simulink model "volo_agcdc_pipelined"  (R2012b)
settings: Solver=ode45  StartTime=0.0  StopTime=1000  RelTol=1e-3
PreLoadFcn:
  | volo_agcdc_init
InitFcn:
  | volo_agcdc_init
StartFcn:
  | volo_agcdc_init
values from neighbouring files (symbols this model uses):
  agc_idleState = 0    [volo_agcdc_init.m]
  agc_numAddrBits = agc_numOutputs + agc_numStateBits    [volo_agcdc_init.m]
  regDCRemoval_AvgLength = 64    [volo_agcdc_init.m]
  regSatDet_NumSamples = 16    [volo_agcdc_init.m]
undefined symbols (not defined in the file or in its folder): gcbh, xlBlockLoadCallback, xlGetNormalizedPeriod
libraries: xbsIndex_r4 x681, xbsEDKLib_r4 x1
(part 5 of 7)

== system volo_agcdc_pipelined/Ext_PktDet_Delay ==
  Set : Inport
  Rst : Inport  Port=2
  "Ext Pkt Det Delay " : Subsystem
  S-R Latch2 : Subsystem
  Out : Outport
  wires:
  S-R Latch2/1(Q) -> "Ext Pkt Det Delay "/1(In)  "ext detect pending"
  Rst/1 -> S-R Latch2/2(R)
  Set/1 -> S-R Latch2/1(S)
  "Ext Pkt Det Delay "/1(Out) -> Out/1  "xternal detection"

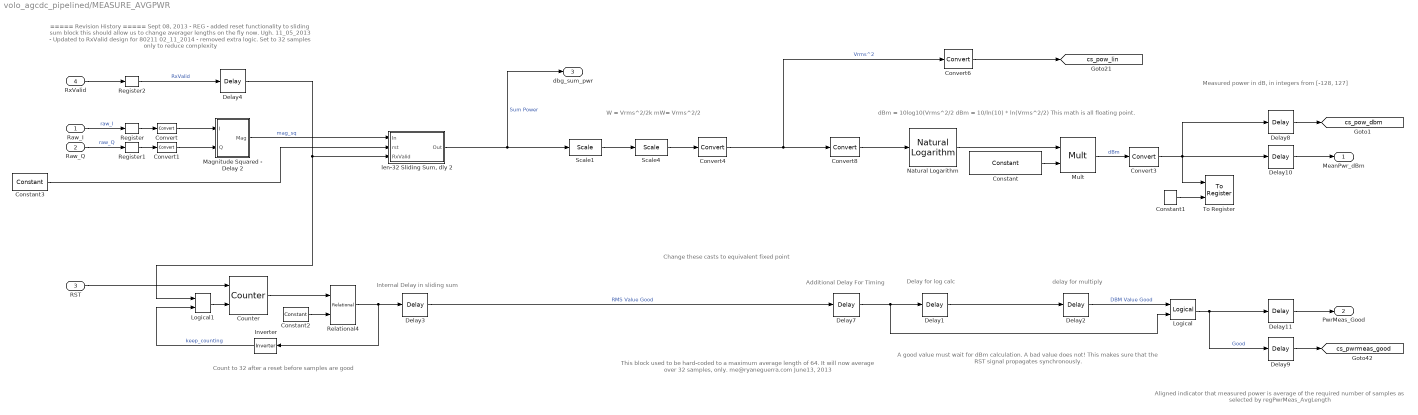
== system volo_agcdc_pipelined/MEASURE_AVGPWR ==
  note: delay for multiply
  note: Delay for log calc
  note: Count to 32 after a reset before samples are good
  note: Change these casts to equivalent fixed point
  note: Additional Delay For Timing
  note: Internal Delay in sliding sum
  note: ===== Revision History =====
      | Sept 08, 2013 - REG - added reset functionality to sliding sum block
      | this should allow us to change averager lengths on the fly now. Ugh.
      | 11_05_2013 - Updated to RxValid design for 80211
      | 02_11_2014 - removed extra logic. Set to 32 samples only to reduce complexity
  note: A good value must wait for dBm calculation.
      | A bad value does not! This makes sure that
      | the RST signal propagates synchronously.
  note: Aligned indicator that
      | measured power is average
      | of the required number
      | of samples as selected
      | by regPwrMeas_AvgLength
  note: Measured power in dB,
      | in  integers from
      | [-128, 127]
  note: dBm = 10log10(Vrms^2/2
      | dBm = 10/ln(10) * ln(Vrms^2/2)
      | This math is all floating point.
  note: W = Vrms^2/2k
      | mW= Vrms^2/2
  note: This block used to be hard-coded to a maximum average length of 64.
      | It will now average over 32 samples, only.
      | me@ryaneguerra.com
      | June13, 2013
  Raw_I : Inport
  Raw_Q : Inport  Port=2
  RST : Inport  Port=3
  RxValid : Inport  Port=4
  Constant : xbsIndex_r4/Constant  const=10/log(10)  gui_display_data_type=Floating-point  arith_type=Floating-point  n_bits=18  bin_pt=14  preci_type=Single  exp_width=8  frac_width=24  explicit_period=on  period=1  equ=P=C  opselect=C  inp2=PCIN>>17  opr=+  inp1=P  carry=CIN  dbl_ovrd=off  block_type=constant
  Constant1 : xbsIndex_r4/Constant  const=1  gui_display_data_type=Boolean  arith_type=Boolean  n_bits=18  bin_pt=14  preci_type=Single  exp_width=8  frac_width=24  explicit_period=on  period=1  equ=P=C  opselect=C  inp2=PCIN>>17  opr=+  inp1=P  carry=CIN  dbl_ovrd=off  block_type=constant
  Constant2 : xbsIndex_r4/Constant  const=32  gui_display_data_type=Fixed-point  arith_type=Unsigned  n_bits=6  bin_pt=0  preci_type=Single  exp_width=8  frac_width=24  explicit_period=on  period=1  equ=P=C  opselect=C  inp2=PCIN>>17  opr=+  inp1=P  carry=CIN  dbl_ovrd=off  block_type=constant
  Constant3 : xbsIndex_r4/Constant  const=0  gui_display_data_type=Boolean  arith_type=Boolean  n_bits=16  bin_pt=14  preci_type=Single  exp_width=8  frac_width=24  explicit_period=on  period=1  equ=P=C  opselect=C  inp2=PCIN>>17  opr=+  inp1=P  carry=CIN  dbl_ovrd=off  block_type=constant
  Convert : xbsIndex_r4/Convert  gui_display_data_type=Fixed-point  arith_type="Signed  (2's comp)"  n_bits=12  bin_pt=11  float_type=Single  exp_bits=8  fraction_bits=24  quantization=Truncate  overflow=Wrap  en=off  latency=0  dbl_ovrd=off  pipeline=off  block_type=convert
  Convert1 : xbsIndex_r4/Convert  gui_display_data_type=Fixed-point  arith_type="Signed  (2's comp)"  n_bits=12  bin_pt=11  float_type=Single  exp_bits=8  fraction_bits=24  quantization=Truncate  overflow=Wrap  en=off  latency=0  dbl_ovrd=off  pipeline=off  block_type=convert
  Convert3 : xbsIndex_r4/Convert  gui_display_data_type=Fixed-point  arith_type="Signed  (2's comp)"  n_bits=9  bin_pt=0  float_type=Single  exp_bits=8  fraction_bits=24  quantization="Round  (unbiased: +/- Inf)"  overflow=Saturate  en=off  latency=0  dbl_ovrd=off  pipeline=off  block_type=convert
  Convert4 : xbsIndex_r4/Convert  gui_display_data_type=Fixed-point  arith_type="Signed  (2's comp)"  n_bits=34  bin_pt=22  float_type=Single  exp_bits=8  fraction_bits=24  quantization=Truncate  overflow=Wrap  en=off  latency=0  dbl_ovrd=off  pipeline=off  block_type=convert
  Convert6 : xbsIndex_r4/Convert  gui_display_data_type=Fixed-point  arith_type="Signed  (2's comp)"  n_bits=32  bin_pt=15  float_type=Single  exp_bits=8  fraction_bits=24  quantization="Round  (unbiased: +/- Inf)"  overflow=Saturate  en=off  latency=0  dbl_ovrd=off  pipeline=off  block_type=convert
  Convert8 : xbsIndex_r4/Convert  gui_display_data_type=Floating-point  arith_type=Floating-point  n_bits=34  bin_pt=22  float_type=Single  exp_bits=8  fraction_bits=24  quantization=Truncate  overflow=Wrap  en=off  latency=3  dbl_ovrd=off  pipeline=on  block_type=convert
  Counter : xbsIndex_r4/Counter  cnt_type=Free Running  cnt_to=10  operation=Up  start_count=0  cnt_by_val=1  arith_type=Unsigned  n_bits=10  bin_pt=0  load_pin=off  rst=on  en=on  explicit_period=on  period=1  dbl_ovrd=off  use_behavioral_HDL=off  implementation=Fabric  block_type=counter
  Delay1 : xbsIndex_r4/Delay  rst=off  infoeditControl=Selection of Reset will increase slice count due to use of real FFs and instead of SRLs  en=off  latency=6  dbl_ovrd=off  reg_retiming=off  block_type=delay
  Delay{8..11} (4 alike) : xbsIndex_r4/Delay  rst=off  infoeditControl=Selection of Reset will increase slice count due to use of real FFs and instead of SRLs  en=off  latency=1  dbl_ovrd=off  reg_retiming=off  block_type=delay
  Delay2 : xbsIndex_r4/Delay  rst=off  infoeditControl=Selection of Reset will increase slice count due to use of real FFs and instead of SRLs  en=off  latency=6  dbl_ovrd=off  reg_retiming=off  block_type=delay
  Delay3 : xbsIndex_r4/Delay  rst=off  infoeditControl=Selection of Reset will increase slice count due to use of real FFs and instead of SRLs  en=off  latency=2  dbl_ovrd=off  reg_retiming=off  block_type=delay
  Delay4 : xbsIndex_r4/Delay  rst=off  infoeditControl=Selection of Reset will increase slice count due to use of real FFs and instead of SRLs  en=off  latency=2  dbl_ovrd=off  reg_retiming=off  block_type=delay
  Delay7 : xbsIndex_r4/Delay  rst=off  infoeditControl=Selection of Reset will increase slice count due to use of real FFs and instead of SRLs  en=off  latency=3  dbl_ovrd=off  reg_retiming=off  block_type=delay
  Inverter : xbsIndex_r4/Inverter  en=off  latency=0  dbl_ovrd=off  block_type=inv
  Logical : xbsIndex_r4/Logical  logical_function=AND  inputs=2  en=off  latency=0  precision=Full  arith_type=Unsigned  n_bits=16  bin_pt=0  align_bp=on  dbl_ovrd=off  block_type=logical
  Logical1 : xbsIndex_r4/Logical  logical_function=AND  inputs=2  en=off  latency=0  precision=Full  arith_type=Unsigned  n_bits=16  bin_pt=0  align_bp=on  dbl_ovrd=off  block_type=logical
  Magnitude Squared - Delay 2 : Subsystem
  Mult : xbsIndex_r4/Mult  precision=Full  arith_type="Signed  (2's comp)"  n_bits=8  bin_pt=0  quantization=Truncate  overflow=Saturate  en=off  latency=6  dbl_ovrd=off  use_behavioral_HDL=off  opt=Speed  use_embedded=on  optimum_pipeline=off  pipeline=on  use_rpm=on  placement_style=Triangular  block_type=mult
  Natural Logarithm : xbsIndex_r4/Natural Logarithm  flow_control=NonBlocking  axi_optimize_goal=Resources  latency=6  has_a_tlast=off  has_a_tuser=off  en=off  has_result_tready=off  has_invalid_op=off  has_divide_by_zero=off  fpo_op_type=log_base_e  rate=1  has_b_tlast=false  has_b_tuser=false  result_tlast_behv=1  has_underflow=false  has_overflow=false  block_type=natlog
      settings: infoedit=Blocking: Wait for data on all inputs, allow back-pressure.<br>NonBlocking: operate every cycle in which all inputs are valid, no back-pressure.
  Register : xbsIndex_r4/Register  init=0  rst=off  en=off  dbl_ovrd=off  block_type=register
  Register1 : xbsIndex_r4/Register  init=0  rst=off  en=off  dbl_ovrd=off  block_type=register
  Register2 : xbsIndex_r4/Register  init=0  rst=off  en=off  dbl_ovrd=off  block_type=register
  Relational4 : xbsIndex_r4/Relational  mode=a=b  en=off  latency=0  dbl_ovrd=off  block_type=relational
  Scale1 : xbsIndex_r4/Scale  scale_factor=-5  dbl_ovrd=off  block_type=scale
  Scale4 : xbsIndex_r4/Scale  scale_factor=-1  dbl_ovrd=off  block_type=scale
  To Register : xbsIndex_r4/To Register  shared_memory_name='regWSD_meanPower'  init=0  ownership=Locally owned and initialized  explicit_data_type=on  gui_display_data_type=Fixed-point  arith_type="Signed  (2's comp)"  n_bits=9  bin_pt=0  preci_type=Single  dbl_ovrd=off  block_type=toreg
      settings: AttributesFormatString=<< %<shared_memory_name> >>  infoedit="Register block that writes data to a shared memory register.  Delay of one sample period."
  "len-32 Sliding Sum, dly 2" : Subsystem
  MeanPwr_dBm : Outport
  PwrMeas_Good : Outport  Port=2
  dbg_sum_pwr : Outport  Port=3
  tag scope: cs_pow_dbm=global, cs_pow_lin=global, cs_pwrmeas_good=global
  wires:
  Magnitude Squared - Delay 2/1(Mag) -> "len-32 Sliding Sum, dly 2"/1(In)  "mag_sq"
  "len-32 Sliding Sum, dly 2"/1(Out) -> dbg_sum_pwr/1, Scale1/1  "Sum Power"
  Raw_I/1 -> Register/1  "raw_I"
  Raw_Q/1 -> Register1/1  "raw_Q"
  Relational4/1 -> Delay3/1, Inverter/1
  Counter/1 -> Relational4/1
  Inverter/1 -> Logical1/2  "keep_counting"
  Convert/1 -> Magnitude Squared - Delay 2/1(I)
  Convert1/1 -> Magnitude Squared - Delay 2/2(Q)
  Convert4/1 -> Convert8/1, Convert6/1  "Vrms^2"
  Natural Logarithm/1 -> Mult/1
  Constant/1 -> Mult/2
  Mult/1 -> Convert3/1  "dBm"
  Convert3/1 -> Delay10/1, Delay8/1, To Register/1
  Delay2/1 -> Logical/1  "DBM Value Good"
  Logical/1 -> Delay11/1, Delay9/1  "Good"
  Scale1/1 -> Scale4/1
  Scale4/1 -> Convert4/1
  Convert6/1 -> [cs_pow_lin]
  Constant3/1 -> "len-32 Sliding Sum, dly 2"/2(rst)
  Constant1/1 -> To Register/2
  Register/1 -> Convert/1
  Register1/1 -> Convert1/1
  RST/1 -> Counter/1
  RxValid/1 -> Register2/1
  Register2/1 -> Delay4/1  "RxValid"
  Logical1/1 -> Counter/2
  Delay1/1 -> Delay2/1
  Delay3/1 -> Delay7/1  "RMS Value Good"
  Convert8/1 -> Natural Logarithm/1
  Delay7/1 -> Logical/2, Delay1/1
  Delay8/1 -> [cs_pow_dbm]
  Delay9/1 -> [cs_pwrmeas_good]
  Delay10/1 -> MeanPwr_dBm/1
  Delay11/1 -> PwrMeas_Good/1
  Constant2/1 -> Relational4/2
  Delay4/1 -> Logical1/1, "len-32 Sliding Sum, dly 2"/3(RxValid)

== system volo_agcdc_pipelined/Measurement Reset Controller ==
  note: When the FSM_Reset signal is active, the OFDM reference model pkt detect is reset.
      | Unfortunately, that signal takes time to propagate through our logic to mask the PwrDet_Good signal.
      | This appears to result in erroneous threshold/delta power detection, so we explicitly and quickly reset the
      | PwrDet and SatDet blocks when the FSM_Reset signal is asserted.
  note: June 21, 2013
      | me@ryaneguerra.com
  SatDet_Rst : Inport
  GainSetBusy : Inport  Port=2
  PwrMeas_Rst : Inport  Port=3
  FSM_Reset : Inport  Port=4
  Logical1 : xbsIndex_r4/Logical  logical_function=OR  inputs=3  en=off  latency=0  precision=Full  arith_type=Unsigned  n_bits=16  bin_pt=0  align_bp=on  dbl_ovrd=off  block_type=logical
  Logical2 : xbsIndex_r4/Logical  logical_function=OR  inputs=3  en=off  latency=0  precision=Full  arith_type=Unsigned  n_bits=16  bin_pt=0  align_bp=on  dbl_ovrd=off  block_type=logical
  SatDetRst_Master : Outport
  PwrMeasRst_Master : Outport  Port=2
  wires:
  GainSetBusy/1 -> Logical1/1, Logical2/2  "Setting Gains"
  PwrMeas_Rst/1 -> Logical1/2  "Explicit PwrMeas Reset"
  SatDet_Rst/1 -> Logical2/1  "Explicit SatDet Reset"
  Logical1/1 -> PwrMeasRst_Master/1
  Logical2/1 -> SatDetRst_Master/1
  FSM_Reset/1 -> Logical1/3, Logical2/3  "Master Reset"

== system volo_agcdc_pipelined/Older Revision Notes ==
  note: January 17, 2014 - 4.03.z - Noticed timing error bug. There was a lot of handoff and mods on
      | this core by others before me. I added a few more registers to be safe. REG
      | January 19, 2014 - 7.00.a - Removed chipscope--too much logic
      | January 19, 2014 - 7.00.b - Addd additional pipelining REG
      | Feb 11, 2014 - 7.00.c - Simplified pwr det and Chipscope. Enabled Chipscope.
      | Fixxed precision issue. REG
      | Feb 13, 2014 - 7.00.d - removed ChipScope. Timing will NOT close with it in. Fuuuuuuu. REG
      | Feb 13, 2014 - 7.00.e - added it back in becasue I'm a badass like that. Edgy REG
      | Feb 25, 2014 - 7.00.f - reworked ChipScope to get RawIQ back in the mix. REG
      | Feb 25, 2014 - 7.00.h - Added input ports for debugging data lines. REG
      | Feb 28, 2014 - 7.00.j - Removed extra port to meet timing. REG
      | March 01, 2014 - 7.00.k - remove DC removal reset port (unused), expanded chipscope, added
      | some debug input ports REG
      | March 1, 2014 - 7.00.m - Removed packet detect HOLD logic because this is WRONG in the
      | 0p8 reference design now. io90pdrfewq=p-o093o09[iCXZ ,mn. REG
      | March 1, 2014 - 7.00.n - Apparently there was a version conflict where I forgot to increment version?
      | Made this version just to prevent any uncertainty as to what was what, REG
      | March 2, 2014 - 7.00.o - Fixed pkt detect loop with Mango Logic. Now all of our local packet
      | detection signals go to the Mango core. The Mango core aggregates packet detection decisions and
      | and that output is sent to the VOLO AGCDC block to trigger AGC.
      | March 2, 2014 - 7.00.p - Added anti-debouncer REG
      | March 5, 2014 - 7.00.q - Completed reset to anti-debouncer. So tired... REG
      | March 13, 2014 - 7.00.r - Ongoing Revision. Pipelining on DC removal block Chipscope Removed. REG
      | March 18, 2014 - 7.00.s - Cleaned up some stuff, added a few pipeline registers to sync with Naren's
      | design. REG
      | MArch 18, 2014 - 7.00.t - MOAR pipelining REG
      | March 30, 2014 - 7.00.u - adjusted DC averaging block and regenerated to update chipscope,
      | which is currently buggy.  REG
      | April 08, 2014 - 7.00.v - added regWSD_RXGAIN_READ reg and moved RSSI latch trigger to
      | LTS_SYNC_2 trigger rather than PayloadGood. Also added SW trigger for gain latch. REG
      | April 23, 2014 - 7.00.w - Re added the external pkt det delay register and one shot timer for WARPLab integration
      | April 29, 2014 - 7.00.x - Added delay to RSSI for Warplab output to ease timing
      | May 21, 2014 - 7.00.y - Modified ChipScope to store post-filter IQ samples. REG
      | May 23, 2014 - 7.00.z - WOW! EDK Processor was creating duplicate register offset addresses.
      | This was the problem that was borking everything. NOTE: it is still not fixed, but we have gone and
      | hand-edited the MPD file with unique, non-overlapping offsets for the To/From registers. REG
  note: Nov 14 2013 - 4.02.p - Setting gain resets the DC removal blockm to avoid
      | stale DC-offset correction values. It's a little slow to correct itself a this time. REG
      | Nov 14, 2013 - 4.02.q - Oops, the last fix was buggy. Also, added a flag to en/dis this reset flag, just
      | in case it proves to not be as great an idea as I hope it is. REG
      | Nov 21, 2013 - 4.02.r - Changed mean_pwr_dbm to correct range for WARPLab
      | Nov 22, 2013 - 4.02.s - Added ExtPktDet_DelayCount register for delaying WARPLab trigger
      | Dec 2, 2013 - 4.02.t - Modified filt_IQ input ports to record post-decimation filter samples REG
      | Dec 10, 2013 - 4.02.u - Added ability to disable minimum power threhsold for autocorrelator. Also
      | increased resolution of autocorr minimum power threshold. REG
      | Dec 11, 2013 - 4.02.v - Allowed deactivation of timeout reset of AGC. This was a bad idea from
      | an old design anyway, but it makes this block not universally useful.
      | Dec 17, 2013 - 4.02.w - Commented out Chipscope REG
  note: Oct 30, 2013 - 0 4.02.a - Changed input/output sampling prec for 802.11 design,
      | changed to AXI bus for EDK, made local autocorr length adjustable
      | Nov 01. 2013 - 4.02.b - Changed autocorrelator block. REG
      | Nov 02, 2013 - 4.02.c - Changed SPITimingFudge Reg and LTS Timeout Counter
      | num bits
      | Nov 02, 2013 - 4.02.d - Added regAGC_InvertHWSPIEndianess option to correct SPI
      | Nov 04, 2013 - 4.02.e - Re-enabled Chipscope
      | Nov 04, 2013 - 4.02.f - Fixed AutoCorrelation block (NOT)
      | Nov 05, 2013 - 4.02.g - Stole Mango80211 Autocorr block, updated SatDet,
      | DC Removal, Energy Detect, Measure AvgPwr to RxValid-based design to
      | allow multiple input sample clock rates while running master clock at
      | 160 MHz. Added Sample Clock Selection block to give software control of sample
      | clock rate. Added PAUSE_AGC input port. REG
      | Nov 06, 2013 - 4.02.h - SPI write GO is now held 8 clock in order to synchronize with
      | slower radio controller clocks that miss the pulse. REG
      | Nov 08 2013 - 4.02.j - filt_I/Q_in are now 12_11; increased length of DC avg block
      | Nov 09 2013 - 4.02.k - Longer Chipscope w/ fewer signals.
      | Nov 13 2013 - 4.02.m - Shorter Chipscope w/ more signals.
      | Nov 13, 2013 - 4.02.n - Added regAGC_WSD_CCAThreshold_dBm to generate CCA for
      | new output port WSD_CCA. Also added WSD_MASK_WARP_PKT_DET port. REG
      | Nov 14, 2013 - 4.02.o - Adjusted ChipScope for LTS info REG
  note: ===== Revision Notes =====
      | Aug 07 2013 - 4.00.a - revert to NOLA IP version, add RSSI reg and port
      | Aug 12, 2013 - 4.00.b - added hard registers for WARPLab gain ctrl when
      | AGC is inactive; this is reqd. because RSSI block needs to know current
      | gain settings.
      | Aug 13, 2013 - 4.00.c - made RX gain registers shared registers for uC access
      | August 15, 2013 - 4.00.d - consolidated shared control register, added packet detect
      | enable signals, added AGC enable signal for direct software gain control
      | August 16, 2013 - 4.00.e - added new register for DynBackoffGain settings, allowed
      | disabling of external packet detect signals from triggering AGCDC AGC.
      | August 16, 2013 - 4.00.f - make regWSD_DynDefaultGain a shared register to monitor
      | background noise levels and also how DynAGCAdaptation is behaving.
      | August 27, 2013 - 4.00.g - Added saturation detection triggers to packet detection, sw_rst
      | for saturation detection, and also made the saturation detection a shared register for sw use
      | September 08, 2013 - 4.00.h - added asynchronous sw-controlled reset to the sliding window
      | on the power averager block. This fixes a bug whereby we couldn't change to 16 or 64 samples
      | because the ASR/Accumulator wouldn't be flushed properly. Now you change LEN, then hold
      | the averager in reset via software for LEN samples.
      | September 09, 2013 - 4.00.i - added the DynDefTrigger to let AGC gain writes and DynDef Gain
      | writes to be enabled/disabled separately.
      | Sept 09, 2013 - 4.00.k - exported the mean measured power as a shared register:
      | regWSD_meanPower
      | Oct 13, 2013 - 4.00.m - fixed weird error (I think) where the FSM_Enable input to the
      | AGC_GAIN_SELECTION block was actually ResetFSM. That's strange, because it means the
      | background adaptation probably wasn't working correctly. Oh shit. We'll see.
      | OCt 15, 2013 - 4.00.o - Updated dynamic holdoff timer with correct(er) logic; added bounds checking REG
      | Oct 16, 2013 - 4.01.a - imported autocorr block from OFDM design, repaired signal definitions for
      | raw/interpolation_filtered/dc-removed, added shared registers to measure mean I/Q, AutoCorr values,
      | and to select AutoCorr parameters and what input is being autocorr'ed.
      | Oct 23, 2013 - 4.01.b - Added EnableFSMResetGainWrite to provide software control over whether
      | or not a reset of the FSM (read: when PktDet goes low due to finished or missed packet)
      | writes current gain settings (meant to reset to default gain after AGC). Also updated signal
      | path for DynTrigger Gain Write signal since it wasn't properly masked. REG
      | Oct 23, 2013 - 4.01.c - Fixed bounds checking--DOH! REG
      | Oct 24, 2013 - 4.01.d - Made DynDefault increase and decrease registers. REG
      | Oct 24, 2013 - 4.01.e - Resynthesis with full ChipScope.
      | Oct 24, 2013 - 4.01.h - Added WSD_AGC_EN_FSMRESETGAINWRITE capability to DynDef block REG
      | Oct 28, 2013 - 4.01.j - Added long_corr_in port and added to chipscope REG
      | Oct 28, 2013 - 4.01.k - Commented out Chipscope.

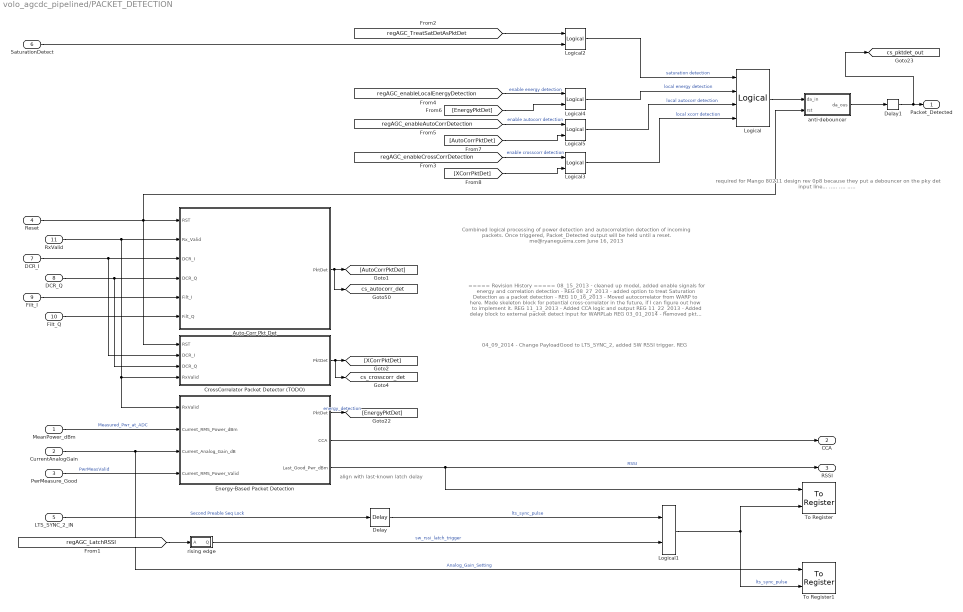
== system volo_agcdc_pipelined/PACKET_DETECTION ==
  note: 04_09_2014 - Change PayloadGood to LTS_SYNC_2, added SW RSSI trigger. REG
  note: required for Mango 80211 design
      | rev 0p8 because they put a debouncer
      | on the pky det input line...
      | .....
      | ....
      | .....
  note: ===== Revision History =====
      | 08_15_2013 - cleaned up model, added enable signals for energy
      | and correlation detection - REG
      | 08_27_2013 - added option to treat Saturation Detection as a packet
      | detection - REG
      | 10_16_2013 - Moved autocorrelator from WARP to here. Made skeleton block
      | for potential cross-correlator in the future, if I can figure out how to implement it. REG
      | 11_13_2013 - Added CCA logic and output REG
      | 11_22_2013 - Added delay block to external packet detect input for WARPLab REG
      | 03_01_2014 - Removed pkt detect hold logic. This is not correct in the 0p8 design anymore. REG
      | 03/02/2014 - added counter-debouncer REG
  note: Combined logical processing of power detection and
      | autocorrelation detection of incoming packets. Once triggered,
      | Packet_Detected output will be held until a reset.
      | me@ryaneguerra.com
      | June 16, 2013
  note: align with last-known
      | latch delay
  MeanPower_dBm : Inport
  CurrentAnalogGain : Inport  Port=2
  PwrMeasure_Good : Inport  Port=3
  Reset : Inport  Port=4
  LTS_SYNC_2_IN : Inport  Port=5
  SaturationDetect : Inport  Port=6
  DCR_I : Inport  Port=7
  DCR_Q : Inport  Port=8
  Filt_I : Inport  Port=9
  Filt_Q : Inport  Port=10
  RxValid : Inport  Port=11
  Auto-Corr Pkt Det : Subsystem
  CrossCorrelator Packet Detector (TODO) : Subsystem
  Delay : xbsIndex_r4/Delay  rst=off  infoeditControl=Selection of Reset will increase slice count due to use of real FFs and instead of SRLs  en=off  latency=1  dbl_ovrd=off  reg_retiming=off  block_type=delay
  Delay1 : xbsIndex_r4/Delay  rst=off  infoeditControl=Selection of Reset will increase slice count due to use of real FFs and instead of SRLs  en=off  latency=1  dbl_ovrd=off  reg_retiming=off  block_type=delay
  Energy-Based Packet Detection : Subsystem
  Logical : xbsIndex_r4/Logical  logical_function=OR  inputs=4  en=off  latency=0  precision=Full  arith_type=Unsigned  n_bits=16  bin_pt=0  align_bp=on  dbl_ovrd=off  block_type=logical
  Logical1 : xbsIndex_r4/Logical  logical_function=OR  inputs=2  en=off  latency=0  precision=Full  arith_type=Unsigned  n_bits=16  bin_pt=0  align_bp=on  dbl_ovrd=off  block_type=logical
  Logical{2..5} (4 alike) : xbsIndex_r4/Logical  logical_function=AND  inputs=2  en=off  latency=0  precision=Full  arith_type=Unsigned  n_bits=16  bin_pt=0  align_bp=on  dbl_ovrd=off  block_type=logical
  To Register : xbsIndex_r4/To Register  shared_memory_name='regWSD_RSSI'  init=0  ownership=Locally owned and initialized  explicit_data_type=on  gui_display_data_type=Fixed-point  arith_type="Signed  (2's comp)"  n_bits=10  bin_pt=0  preci_type=Single  dbl_ovrd=off  block_type=toreg
      settings: AttributesFormatString=<< %<shared_memory_name> >>  infoedit="Register block that writes data to a shared memory register.  Delay of one sample period."
  To Register1 : xbsIndex_r4/To Register  shared_memory_name='regWSD_RXGAIN_READ'  init=0  ownership=Locally owned and initialized  explicit_data_type=on  gui_display_data_type=Fixed-point  arith_type="Signed  (2's comp)"  n_bits=9  bin_pt=0  preci_type=Single  dbl_ovrd=off  block_type=toreg
      settings: AttributesFormatString=<< %<shared_memory_name> >>  infoedit="Register block that writes data to a shared memory register.  Delay of one sample period."
  anti-debouncer : Subsystem
  rising edge : Subsystem
  Packet_Detected : Outport
  CCA : Outport  Port=2
  RSSI : Outport  Port=3
  tag scope: cs_autocorr_det=global, cs_crosscorr_det=global, cs_pktdet_out=global
  wires:
  Reset/1 -> anti-debouncer/2(rst), CrossCorrelator Packet Detector (TODO)/1(RST), Auto-Corr Pkt Det/1(RST)
  PwrMeasure_Good/1 -> Energy-Based Packet Detection/4(Current_RMS_Power_Valid)  "PwrMeasValid"
  LTS_SYNC_2_IN/1 -> Delay/1  "Second Preable Seq Lock"
  Logical1/1 -> To Register/2, To Register1/2  "lts_sync_pulse"
  Logical4/1 -> Logical/2  "local energy detection"
  [regAGC_enableLocalEnergyDetection] -> Logical4/1  "enable energy detection"
  Logical5/1 -> Logical/3  "local autocorr detection"
  [regAGC_enableAutoCorrDetection] -> Logical5/1  "enable autocorr detection"
  MeanPower_dBm/1 -> Energy-Based Packet Detection/2(Current_RMS_Power_dBm)  "Measured_Pwr_at_ADC"
  CurrentAnalogGain/1 -> To Register1/1, Energy-Based Packet Detection/3(Current_Analog_Gain_dB)  "Analog_Gain_Setting"
  [regAGC_TreatSatDetAsPktDet] -> Logical2/1
  SaturationDetect/1 -> Logical2/2
  Logical2/1 -> Logical/1  "saturation detection"
  [regAGC_enableCrossCorrDetection] -> Logical3/1  "enable crosscorr detection"
  Energy-Based Packet Detection/1(PktDet) -> [EnergyPktDet]  "energy_detection"
  [EnergyPktDet] -> Logical4/2
  [XCorrPktDet] -> Logical3/2
  [AutoCorrPktDet] -> Logical5/2
  Logical3/1 -> Logical/4  "local xcorr detection"
  DCR_Q/1 -> CrossCorrelator Packet Detector (TODO)/3(DCR_Q), Auto-Corr Pkt Det/4(DCR_Q)
  DCR_I/1 -> CrossCorrelator Packet Detector (TODO)/2(DCR_I), Auto-Corr Pkt Det/3(DCR_I)
  Filt_I/1 -> Auto-Corr Pkt Det/5(Filt_I)
  Filt_Q/1 -> Auto-Corr Pkt Det/6(Filt_Q)
  Auto-Corr Pkt Det/1(PktDet) -> [AutoCorrPktDet], [cs_autocorr_det]
  CrossCorrelator Packet Detector (TODO)/1(PktDet) -> [XCorrPktDet], [cs_crosscorr_det]
  Energy-Based Packet Detection/3(Last_Good_Pwr_dBm) -> RSSI/1, To Register/1  "RSSI"
  RxValid/1 -> Energy-Based Packet Detection/1(RxValid), CrossCorrelator Packet Detector (TODO)/4(RxValid), Auto-Corr Pkt Det/2(Rx_Valid)
  Energy-Based Packet Detection/2(CCA) -> CCA/1
  anti-debouncer/1(da_ous) -> Delay1/1
  Delay1/1 -> [cs_pktdet_out], Packet_Detected/1
  Logical/1 -> anti-debouncer/1(da_in)
  [regAGC_LatchRSSI] -> rising edge/1(A)
  rising edge/1(Q) -> Logical1/2  "sw_rssi_latch_trigger"
  Delay/1 -> Logical1/1  "lts_sync_pulse"

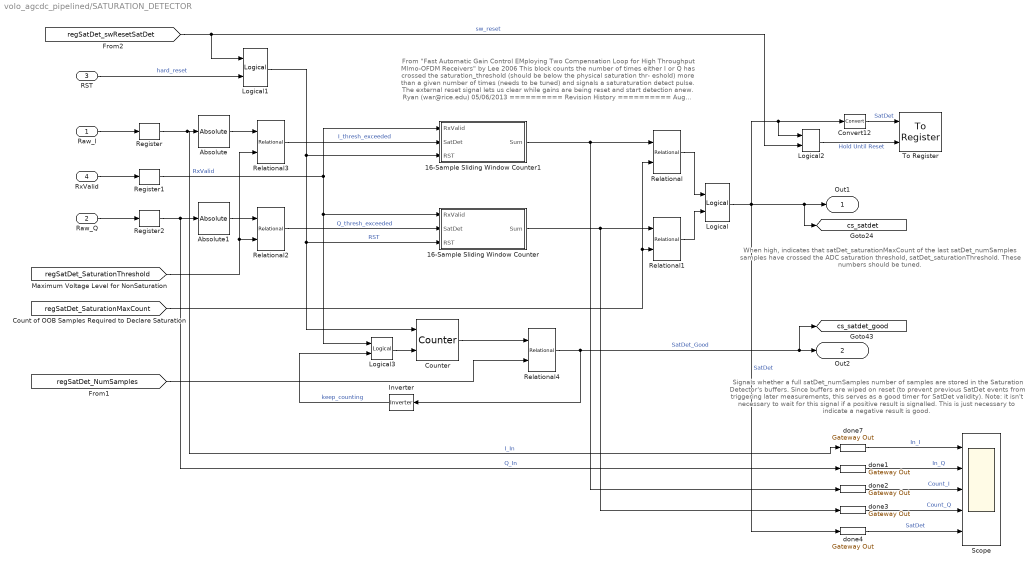
== system volo_agcdc_pipelined/SATURATION_DETECTOR ==
  note: When high, indicates that satDet_saturationMaxCount of the last
      | satDet_numSamples samples have crossed the ADC saturation threshold,
      | satDet_saturationThreshold. These numbers should be tuned.
  note: Signals whether a full satDet_numSamples number of samples
      | are stored in the Saturation Detector's buffers. Since buffers are
      | wiped on reset (to prevent previous SatDet events from triggering
      | later measurements, this serves as a good timer for SatDet validity).
      | Note: it isn't necessary to wait for this signal if a positive result is
      | signalled. This is just necessary to indicate a negative result is good.
  note: From "Fast Automatic Gain Control EMploying Two Compensation Loop for High Throughput MImo-OFDM Receivers" by Lee 2006
      | This block counts the number of times either I or Q has crossed the saturation_threshold (should be below the physical saturation thr-
      | eshold) more than a given number of times (needs to be tuned) and signals a saturaturation detect pulse. The external reset signal lets
      | us clear while gains are being reset and start detection anew. Ryan (war@rice.edu) 05/06/2013
      | ==========  Revision History ==========
      | Aug 27, 2013 - added SW_Reset capabilities and output shared register for testing saturation levels with software.
      | 11_5_2013 - Converted to RxValid-based design for 80211 REG
  Raw_I : Inport
  Raw_Q : Inport  Port=2
  RST : Inport  Port=3
  RxValid : Inport  Port=4
  16-Sample Sliding Window Counter : Subsystem
  16-Sample Sliding Window Counter1 : Subsystem
  Absolute : xbsIndex_r4/Absolute  precision=Full  arith_type=Unsigned  n_bits=16  bin_pt=14  quantization=Truncate  overflow=Wrap  en=off  latency=0  dbl_ovrd=off  block_type=abs
  Absolute1 : xbsIndex_r4/Absolute  precision=Full  arith_type=Unsigned  n_bits=16  bin_pt=14  quantization=Truncate  overflow=Wrap  en=off  latency=0  dbl_ovrd=off  block_type=abs
  Convert12 : xbsIndex_r4/Convert  gui_display_data_type=Fixed-point  arith_type=Unsigned  n_bits=1  bin_pt=0  float_type=Single  exp_bits=8  fraction_bits=24  quantization=Truncate  overflow=Wrap  en=off  latency=0  dbl_ovrd=off  pipeline=off  block_type=convert
  Counter : xbsIndex_r4/Counter  cnt_type=Free Running  cnt_to=regSatDet_NumSamples  operation=Up  start_count=0  cnt_by_val=1  arith_type=Unsigned  n_bits=ceil(log(regSatDet_NumSamples)/log(2))+1  bin_pt=0  load_pin=off  rst=on  en=on  explicit_period=on  period=1  dbl_ovrd=off  use_behavioral_HDL=off  implementation=Fabric  block_type=counter
  Inverter : xbsIndex_r4/Inverter  en=off  latency=0  dbl_ovrd=off  block_type=inv
  Logical : xbsIndex_r4/Logical  logical_function=OR  inputs=2  en=off  latency=0  precision=Full  arith_type=Unsigned  n_bits=16  bin_pt=0  align_bp=on  dbl_ovrd=off  block_type=logical
  Logical1 : xbsIndex_r4/Logical  logical_function=OR  inputs=2  en=off  latency=0  precision=Full  arith_type=Unsigned  n_bits=16  bin_pt=0  align_bp=on  dbl_ovrd=off  block_type=logical
  Logical2 : xbsIndex_r4/Logical  logical_function=OR  inputs=2  en=off  latency=0  precision=Full  arith_type=Unsigned  n_bits=16  bin_pt=0  align_bp=on  dbl_ovrd=off  block_type=logical
  Logical3 : xbsIndex_r4/Logical  logical_function=AND  inputs=2  en=off  latency=0  precision=Full  arith_type=Unsigned  n_bits=16  bin_pt=0  align_bp=on  dbl_ovrd=off  block_type=logical
  Register : xbsIndex_r4/Register  init=0  rst=off  en=off  dbl_ovrd=off  block_type=register
  Register1 : xbsIndex_r4/Register  init=0  rst=off  en=off  dbl_ovrd=off  block_type=register
  Register2 : xbsIndex_r4/Register  init=0  rst=off  en=off  dbl_ovrd=off  block_type=register
  Relational{,1..3} (4 alike) : xbsIndex_r4/Relational  mode=a>b  en=off  latency=0  dbl_ovrd=off  block_type=relational
  Relational4 : xbsIndex_r4/Relational  mode=a=b  en=off  latency=0  dbl_ovrd=off  block_type=relational
  Scope : Scope  NumInputPorts=5
      settings: ShowLegends=on  YMin=-5~-5~-5~-5~-5  YMax=5~5~5~5~5  SaveName=ScopeData3
  To Register : xbsIndex_r4/To Register  shared_memory_name='regSatDet_SaturationDetected'  init=0  ownership=Locally owned and initialized  explicit_data_type=on  gui_display_data_type=Fixed-point  arith_type=Unsigned  n_bits=1  bin_pt=0  preci_type=Single  dbl_ovrd=off  block_type=toreg
      settings: AttributesFormatString=<< %<shared_memory_name> >>  infoedit="Register block that writes data to a shared memory register.  Delay of one sample period."
  done{1..4,7} (5 alike) : xbsIndex_r4/Gateway Out  inherit_from_input=off  hdl_port=off  timing_constraint=None  locs_specified=off  LOCs={}  UseAsDAC=off  DACChannel='1'  block_type=gatewayout
      settings: infoedit="Gateway out block.  Converts Xilinx fixed point inputs into ouputs of type Simulink integer, double, or fixed point.<P><P>Hardware notes:  In hardware these blocks become top level output ports or are discarded, depending on how they are configured."  xl_area=[0 0 0 0 1 0 0]  block_version=VER_STRING_GOES_HERE
  Out1 : Outport
  Out2 : Outport  Port=2
  tag scope: cs_satdet=global, cs_satdet_good=global
  wires:
  [regSatDet_SaturationMaxCount] -> Relational1/2, Relational/2
  Relational1/1 -> Logical/2
  Logical/1 -> Convert12/1, Logical2/1, done4/1, [cs_satdet], Out1/1  "SatDet"
  Relational/1 -> Logical/1
  Relational3/1 -> 16-Sample Sliding Window Counter1/2(SatDet)  "I_thresh_exceeded"
  Raw_Q/1 -> Register2/1
  Raw_I/1 -> Register/1
  [regSatDet_SaturationThreshold] -> Relational2/2, Relational3/2
  Logical1/1 -> 16-Sample Sliding Window Counter1/3(RST), Counter/1, 16-Sample Sliding Window Counter/3(RST)  "RST"
  Absolute/1 -> Relational3/1
  Absolute1/1 -> Relational2/1
  done7/1 -> Scope/1  "In_I"
  done1/1 -> Scope/2  "In_Q"
  done2/1 -> Scope/3  "Count_I"
  done3/1 -> Scope/4  "Count_Q"
  done4/1 -> Scope/5  "SatDet"
  16-Sample Sliding Window Counter1/1(Sum) -> done2/1, Relational/1
  Relational4/1 -> [cs_satdet_good], Out2/1, Inverter/1  "SatDet_Good"
  Counter/1 -> Relational4/1
  [regSatDet_NumSamples] -> Relational4/2
  Inverter/1 -> Logical3/2  "keep_counting"
  RST/1 -> Logical1/2  "hard_reset"
  [regSatDet_swResetSatDet] -> Logical2/2, Logical1/1  "sw_reset"
  Logical2/1 -> To Register/2  "Hold Until Reset"
  Convert12/1 -> To Register/1  "SatDet"
  RxValid/1 -> Register1/1
  Register/1 -> done7/1, Absolute/1  "I_In"
  Register1/1 -> 16-Sample Sliding Window Counter1/1(RxValid), 16-Sample Sliding Window Counter/1(RxValid), Logical3/1  "RxValid"
  Register2/1 -> done1/1, Absolute1/1  "Q_In"
  Logical3/1 -> Counter/2
  16-Sample Sliding Window Counter/1(Sum) -> done3/1, Relational1/1
  Relational2/1 -> 16-Sample Sliding Window Counter/2(SatDet)  "Q_thresh_exceeded"

== system volo_agcdc_pipelined/Sample Clock Selection ==
  note: Assuming 160 MHz Clock:
      | 00 = 40 MHz
      | 01 = 20 MHz
      | 10 = 10 MHz
      | 11 = 20 MHz
      |
      | With 80 MHz clock, these rate just divide by two.
  Constant1 : xbsIndex_r4/Constant  const=1  gui_display_data_type=Boolean  arith_type=Boolean  n_bits=16  bin_pt=14  preci_type=Single  exp_width=8  frac_width=24  explicit_period=on  period=8  equ=P=C  opselect=C  inp2=PCIN>>17  opr=+  inp1=P  carry=CIN  dbl_ovrd=off  block_type=constant
  Constant2 : xbsIndex_r4/Constant  const=1  gui_display_data_type=Boolean  arith_type=Boolean  n_bits=16  bin_pt=14  preci_type=Single  exp_width=8  frac_width=24  explicit_period=on  period=16  equ=P=C  opselect=C  inp2=PCIN>>17  opr=+  inp1=P  carry=CIN  dbl_ovrd=off  block_type=constant
  Constant3 : xbsIndex_r4/Constant  const=1  gui_display_data_type=Boolean  arith_type=Boolean  n_bits=16  bin_pt=14  preci_type=Single  exp_width=8  frac_width=24  explicit_period=on  period=32  equ=P=C  opselect=C  inp2=PCIN>>17  opr=+  inp1=P  carry=CIN  dbl_ovrd=off  block_type=constant
  Constant4 : xbsIndex_r4/Constant  const=1  gui_display_data_type=Boolean  arith_type=Boolean  n_bits=16  bin_pt=14  preci_type=Single  exp_width=8  frac_width=24  explicit_period=on  period=4  equ=P=C  opselect=C  inp2=PCIN>>17  opr=+  inp1=P  carry=CIN  dbl_ovrd=off  block_type=constant
  Constant5 : xbsIndex_r4/Constant  const=1  gui_display_data_type=Boolean  arith_type=Boolean  n_bits=16  bin_pt=14  preci_type=Single  exp_width=8  frac_width=24  explicit_period=on  period=2  equ=P=C  opselect=C  inp2=PCIN>>17  opr=+  inp1=P  carry=CIN  dbl_ovrd=off  block_type=constant
  Mux : xbsIndex_r4/Mux  inputs=4  en=off  latency=0  precision=Full  arith_type=Unsigned  n_bits=16  bin_pt=14  quantization=Truncate  overflow=Wrap  dbl_ovrd=off  block_type=mux
  Mux1 : xbsIndex_r4/Mux  inputs=4  en=off  latency=0  precision=Full  arith_type=Unsigned  n_bits=16  bin_pt=14  quantization=Truncate  overflow=Wrap  dbl_ovrd=off  block_type=mux
  Up Sample : xbsIndex_r4/Up Sample  sample_ratio=8  copy_samples=off  en=off  latency=0  dbl_ovrd=off  block_type=usamp
  Up Sample1 : xbsIndex_r4/Up Sample  sample_ratio=16  copy_samples=off  en=off  latency=0  dbl_ovrd=off  block_type=usamp
  Up Sample2 : xbsIndex_r4/Up Sample  sample_ratio=32  copy_samples=off  en=off  latency=0  dbl_ovrd=off  block_type=usamp
  Up Sample3 : xbsIndex_r4/Up Sample  sample_ratio=4  copy_samples=off  en=off  latency=0  dbl_ovrd=off  block_type=usamp
  Up Sample4 : xbsIndex_r4/Up Sample  sample_ratio=2  copy_samples=off  en=off  latency=0  dbl_ovrd=off  block_type=usamp
  OFDMSampleValid : Outport
  SampleValid : Outport  Port=2
  tag scope: cs_rxvalid=global
  wires:
  Constant1/1 -> Up Sample/1
  Constant2/1 -> Up Sample1/1
  Constant3/1 -> Up Sample2/1
  [regAGC_OFDMSampleRateSel] -> Mux/1
  Up Sample/1 -> Mux1/4, Mux/3  "160/8 = 20 MHz"
  Up Sample1/1 -> Mux1/5, Mux/4  "160/16 = 10 MHz"
  Up Sample2/1 -> Mux/5  "160/32 = 5 MHz"
  Mux/1 -> OFDMSampleValid/1, [cs_rxvalid]
  Constant4/1 -> Up Sample3/1
  Up Sample3/1 -> Mux/2, Mux1/3  "160/4 = 40 MHz"
  Constant5/1 -> Up Sample4/1
  Up Sample4/1 -> Mux1/2  "160/2 = 80 MHz"
  Mux1/1 -> SampleValid/1
  [regAGC_SampleRateSel] -> Mux1/1

== system volo_agcdc_pipelined/TOP_LEVEL_AGC_TIMING ==
  note: Modifications
      | 01_18_2014 - Removed the reset counter logic. That functionality should be handled by MAC REG
  note: My apologies for the mess. This block handles some of the top-level timing:
      | 1. Enabling/disabling AGC+PktDetection and resetting the AGC FSM
      | 2. Generating the AGCDone signal when the FSM has finished.
      | me@ryaneguerra.com
  note: When we enter the MeasurePwr state 7
      | and the fine gain step count is maxed, then
      | AGC is done.
  note: note: Pkt_Detect is held until reset
  Pkt_Detect : Inport
  PHY_AGC_Enable : Inport  Port=2
  AGC_Reset : Inport  Port=3
  FSM_State : Inport  Port=4
  PwrSet_Inc : Inport  Port=5
  Constant : xbsIndex_r4/Constant  const=7  gui_display_data_type=Fixed-point  arith_type=Unsigned  n_bits=3  bin_pt=0  preci_type=Single  exp_width=8  frac_width=24  explicit_period=off  period=1  equ=P=C  opselect=C  inp2=PCIN>>17  opr=+  inp1=P  carry=CIN  dbl_ovrd=off  block_type=constant
  HoldUntilReset2 : Subsystem
  Inverter2 : xbsIndex_r4/Inverter  en=off  latency=0  dbl_ovrd=off  block_type=inv
  Logical{1,5..7} (4 alike) : xbsIndex_r4/Logical  logical_function=AND  inputs=2  en=off  latency=0  precision=Full  arith_type=Unsigned  n_bits=16  bin_pt=0  align_bp=on  dbl_ovrd=off  block_type=logical
  Logical4 : xbsIndex_r4/Logical  logical_function=OR  inputs=2  en=off  latency=0  precision=Full  arith_type=Unsigned  n_bits=16  bin_pt=0  align_bp=on  dbl_ovrd=off  block_type=logical
  PayloadTimeoutCounter : xbsIndex_r4/Counter  cnt_type=Free Running  cnt_to=Inf  operation=Up  start_count=0  cnt_by_val=1  arith_type=Unsigned  n_bits=4  bin_pt=0  load_pin=off  rst=on  en=on  explicit_period=on  period=1  dbl_ovrd=off  use_behavioral_HDL=off  implementation=Fabric  block_type=counter
  Relational : xbsIndex_r4/Relational  mode=a=b  en=off  latency=0  dbl_ovrd=off  block_type=relational
  Relational1 : xbsIndex_r4/Relational  mode=a=b  en=off  latency=0  dbl_ovrd=off  block_type=relational
  rising edge : Subsystem
  FSM_Enable : Outport
  Enable_AGC : Outport  Port=2
  ResetAGC : Outport  Port=3
  AGC_Done : Outport  Port=4
  tag scope: cs_agcdone=global, cs_fsm_enable=global, cs_reset_fsm=global
  wires:
  Pkt_Detect/1 -> Logical5/1  "packet detected"
  Logical1/1 -> [cs_fsm_enable], FSM_Enable/1
  Logical7/1 -> Enable_AGC/1, Logical1/2  "RST"
  Logical4/1 -> PayloadTimeoutCounter/1, rising edge/1(A), HoldUntilReset2/2(RST), [cs_reset_fsm], ResetAGC/1
  Logical5/1 -> Logical1/1
  rising edge/1(Q) -> Inverter2/1
  Inverter2/1 -> Logical5/2  "drop low one cycle on reset"
  PwrSet_Inc/1 -> PayloadTimeoutCounter/2
  Relational/1 -> Logical6/2
  [regAGC_NumFineGainSteps] -> Relational/2
  PayloadTimeoutCounter/1 -> Relational/1
  Relational1/1 -> Logical6/1
  Logical6/1 -> HoldUntilReset2/1(A)
  FSM_State/1 -> Relational1/1
  Constant/1 -> Relational1/2
  HoldUntilReset2/1(Q) -> [cs_agcdone], AGC_Done/1
  AGC_Reset/1 -> Logical4/2  "phy reset"
  [regAGC_enableWSDAGC] -> Logical7/1
  PHY_AGC_Enable/1 -> Logical7/2  "RST"
  [regAGC_resetWSDAGC] -> Logical4/1  "soft reset"

== system volo_agcdc_pipelined/AGC Shared Registers/Dynamic Background Adaptation ==
  Bits[0:5] : xbsIndex_r4/Slice  nbits=6  boolean_output=off  mode=Lower Bit Location + Width  bit1=0  base1=MSB of Input  bit0=0  base0=LSB of Input  dbl_ovrd=off  block_type=slice
  Bits[6:11] : xbsIndex_r4/Slice  nbits=6  boolean_output=off  mode=Lower Bit Location + Width  bit1=0  base1=MSB of Input  bit0=6  base0=LSB of Input  dbl_ovrd=off  block_type=slice
  From Register1 : xbsIndex_r4/From Register  shared_memory_name='regAGC_GainStepSizes'  init=3*2^6 + 1*2^0  period=1  ownership=Locally owned and initialized  gui_display_data_type=Fixed-point  arith_type=Unsigned  n_bits=32  bin_pt=0  preci_type=Single  dbl_ovrd=off  block_type=fromreg
      settings: AttributesFormatString=<< %<shared_memory_name> >>  infoedit="Register block that reads data to a shared memory register.  Delay of one sample period."
  From Register15 : xbsIndex_r4/From Register  shared_memory_name='regAGC_DynBackoffSettings'  init=regAGC_DynBackoffSettings  period=1  ownership=Locally owned and initialized  gui_display_data_type=Fixed-point  arith_type=Unsigned  n_bits=32  bin_pt=0  preci_type=Single  dbl_ovrd=off  block_type=fromreg
      settings: AttributesFormatString=<< %<shared_memory_name> >>  infoedit="Register block that reads data to a shared memory register.  Delay of one sample period."
  From Register18 : xbsIndex_r4/From Register  shared_memory_name='regAGC_MaxDynDefaultGain'  init=61  period=1  ownership=Locally owned and initialized  gui_display_data_type=Fixed-point  arith_type=Unsigned  n_bits=6  bin_pt=0  preci_type=Single  dbl_ovrd=off  block_type=fromreg
      settings: AttributesFormatString=<< %<shared_memory_name> >>  infoedit="Register block that reads data to a shared memory register.  Delay of one sample period."
  From Register19 : xbsIndex_r4/From Register  shared_memory_name='regAGC_DynMinimumGain'  init=-25  period=1  ownership=Locally owned and initialized  gui_display_data_type=Fixed-point  arith_type="Signed  (2's comp)"  n_bits=9  bin_pt=0  preci_type=Single  dbl_ovrd=off  block_type=fromreg
      settings: AttributesFormatString=<< %<shared_memory_name> >>  infoedit="Register block that reads data to a shared memory register.  Delay of one sample period."
  From Register20 : xbsIndex_r4/From Register  shared_memory_name='regAGC_DynAdjustmentHoldoffTimer'  init=0  period=1  ownership=Locally owned and initialized  gui_display_data_type=Fixed-point  arith_type=Unsigned  n_bits=32  bin_pt=0  preci_type=Single  dbl_ovrd=off  block_type=fromreg
      settings: AttributesFormatString=<< %<shared_memory_name> >>  infoedit="Register block that reads data to a shared memory register.  Delay of one sample period."
  From Register21 : xbsIndex_r4/From Register  shared_memory_name='regAGC_MinDynDefaultGain'  init=6  period=1  ownership=Locally owned and initialized  gui_display_data_type=Fixed-point  arith_type=Unsigned  n_bits=6  bin_pt=0  preci_type=Single  dbl_ovrd=off  block_type=fromreg
      settings: AttributesFormatString=<< %<shared_memory_name> >>  infoedit="Register block that reads data to a shared memory register.  Delay of one sample period."
  to_u6_0 : xbsIndex_r4/Convert  gui_display_data_type=Fixed-point  arith_type=Unsigned  n_bits=6  bin_pt=0  float_type=Single  exp_bits=8  fraction_bits=24  quantization=Truncate  overflow=Wrap  en=off  latency=0  dbl_ovrd=off  pipeline=off  block_type=convert
  to_u6_1 : xbsIndex_r4/Convert  gui_display_data_type=Fixed-point  arith_type=Unsigned  n_bits=6  bin_pt=0  float_type=Single  exp_bits=8  fraction_bits=24  quantization=Truncate  overflow=Wrap  en=off  latency=0  dbl_ovrd=off  pipeline=off  block_type=convert
  tag scope: regAGC_DynAdjustment_HoldoffTimer=global, regAGC_DynAdjustment_MaxDefaultGain=global, regAGC_DynAdjustment_MinDefaultGain=global, regAGC_DynBackoffSettings=global, regAGC_DynMinimumPwr=global, regAGC_GainDecreaseStep=global, regAGC_GainIncreaseStep=global
  wires:
  From Register19/1 -> [regAGC_DynMinimumPwr]
  From Register20/1 -> [regAGC_DynAdjustment_HoldoffTimer]
  From Register15/1 -> [regAGC_DynBackoffSettings]
  From Register18/1 -> [regAGC_DynAdjustment_MaxDefaultGain]
  From Register21/1 -> [regAGC_DynAdjustment_MinDefaultGain]
  Bits[0:5]/1 -> to_u6_0/1
  Bits[6:11]/1 -> to_u6_1/1
  to_u6_0/1 -> [regAGC_GainIncreaseStep]
  From Register1/1 -> Bits[6:11]/1, Bits[0:5]/1
  to_u6_1/1 -> [regAGC_GainDecreaseStep]

== system volo_agcdc_pipelined/AGC_GAIN_SELECTION/rising edge ==
  note: rising edge
  A : Inport
  Convert : xbsIndex_r4/Convert  gui_display_data_type=Boolean  arith_type=Boolean  n_bits=16  bin_pt=14  float_type=Single  exp_bits=8  fraction_bits=24  quantization=Truncate  overflow=Wrap  en=off  latency=0  dbl_ovrd=off  pipeline=off  block_type=convert
  Delay1 : xbsIndex_r4/Delay  rst=off  infoeditControl=Selection of Reset will increase slice count due to use of real FFs and instead of SRLs  en=off  latency=1  dbl_ovrd=off  reg_retiming=off  block_type=delay
  Inverter2 : xbsIndex_r4/Inverter  en=off  latency=0  dbl_ovrd=off  block_type=inv
  Logical2 : xbsIndex_r4/Logical  logical_function=AND  inputs=2  en=off  latency=0  precision=Full  arith_type=Unsigned  n_bits=16  bin_pt=0  align_bp=on  dbl_ovrd=off  block_type=logical
  Q : Outport
  wires:
  Logical2/1 -> Convert/1
  A/1 -> Logical2/1, Delay1/1
  Delay1/1 -> Inverter2/1
  Inverter2/1 -> Logical2/2
  Convert/1 -> Q/1
